simulink model "dc_motor"  (R2017b)
settings: Solver=VariableStepAuto  StartTime=0.0  StopTime=0.3  RelTol=1e-3
InitFcn:
  | before_simulation
values from neighbouring files (symbols this model uses):
  J = 0.08    [before_simulation.m]
  Kb = 0.87    [before_simulation.m]
  Kf = 0.043    [before_simulation.m]
  Km = 1.34    [before_simulation.m]
  L = 0.05    [before_simulation.m]
  R = 1.7    [before_simulation.m]
libraries: simulink_extras x6, simulink x4
settings Model: Creator=Iman  LastModifiedBy=Iman
settings DataIOCC: SaveFormat=Array

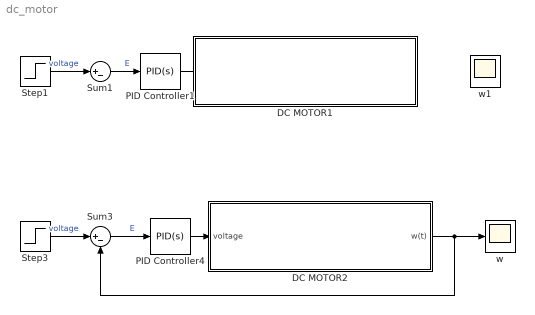
== system dc_motor ==
  DC MOTOR1 : Subsystem
  DC MOTOR2 : Subsystem
  PID Controller1 : simulink/Continuous/PID Controller  Controller=PID  TimeDomain=Continuous-time  SampleTime=-1  IntegratorMethod=Forward Euler  FilterMethod=Forward Euler  Form=Parallel  UseFilter=on  ControllerParametersSource=internal  P=89.3450380919849  I=457.97727460553  D=4.14027320331142  N=464.681776716059  InitialConditionSource=internal  InitialConditionForIntegrator=0  InitialConditionForFilter=0  ExternalReset=none  LimitOutput=off  UpperSaturationLimit=inf  LowerSaturationLimit=-inf  LinearizeAsGain=on  AntiWindupMode=none  Kb=1  TrackingMode=off  Kt=1  PParamMin=[]  PParamMax=[]  IParamMin=[]  IParamMax=[]  DParamMin=[]  DParamMax=[]  NParamMin=[]  NParamMax=[]  KbParamMin=[]  KbParamMax=[]  KtParamMin=[]  KtParamMax=[]  POutMin=[]  POutMax=[]  IOutMin=[]  IOutMax=[]  DOutMin=[]  DOutMax=[]  NOutMin=[]  NOutMax=[]  KbOutMin=[]  KbOutMax=[]  KtOutMin=[]  KtOutMax=[]  IntegratorOutMin=[]  IntegratorOutMax=[]  FilterOutMin=[]  FilterOutMax=[]  SumOutMin=[]  SumOutMax=[]  SumI1OutMin=[]  SumI1OutMax=[]  SumI2OutMin=[]  SumI2OutMax=[]  SumI3OutMin=[]  SumI3OutMax=[]  SumDOutMin=[]  SumDOutMax=[]  SaturationOutMin=[]  SaturationOutMax=[]  IntegratorContinuousStateAttributes=''  IntegratorStateMustResolveToSignalObject=off  IntegratorRTWStateStorageClass=Auto  FilterContinuousStateAttributes=''  FilterStateMustResolveToSignalObject=off  FilterRTWStateStorageClass=Auto  DifferentiatorICPrevScaledInput=0  DifferentiatorOutMin=[]  DifferentiatorOutMax=[]  InitialConditionSetting=State (most efficient)  FilterDiffOutCoefMin=[]  FilterDiffOutCoefMax=[]  SumDenOutMin=[]  SumDenOutMax=[]  SumNumOutMin=[]  SumNumOutMax=[]  ReciprocalOutMin=[]  ReciprocalOutMax=[]  DivideOutMin=[]  DivideOutMax=[]  TunerSelectOption=Transfer Function Based (PID Tuner App)
  PID Controller4 : simulink/Continuous/PID Controller  Controller=PID  TimeDomain=Continuous-time  SampleTime=-1  IntegratorMethod=Forward Euler  FilterMethod=Forward Euler  Form=Parallel  UseFilter=on  ControllerParametersSource=internal  P=89.3450380919849  I=457.97727460553  D=4.14027320331142  N=464.681776716059  InitialConditionSource=internal  InitialConditionForIntegrator=0  InitialConditionForFilter=0  ExternalReset=none  LimitOutput=off  UpperSaturationLimit=inf  LowerSaturationLimit=-inf  LinearizeAsGain=on  AntiWindupMode=none  Kb=1  TrackingMode=off  Kt=1  PParamMin=[]  PParamMax=[]  IParamMin=[]  IParamMax=[]  DParamMin=[]  DParamMax=[]  NParamMin=[]  NParamMax=[]  KbParamMin=[]  KbParamMax=[]  KtParamMin=[]  KtParamMax=[]  POutMin=[]  POutMax=[]  IOutMin=[]  IOutMax=[]  DOutMin=[]  DOutMax=[]  NOutMin=[]  NOutMax=[]  KbOutMin=[]  KbOutMax=[]  KtOutMin=[]  KtOutMax=[]  IntegratorOutMin=[]  IntegratorOutMax=[]  FilterOutMin=[]  FilterOutMax=[]  SumOutMin=[]  SumOutMax=[]  SumI1OutMin=[]  SumI1OutMax=[]  SumI2OutMin=[]  SumI2OutMax=[]  SumI3OutMin=[]  SumI3OutMax=[]  SumDOutMin=[]  SumDOutMax=[]  SaturationOutMin=[]  SaturationOutMax=[]  IntegratorContinuousStateAttributes=''  IntegratorStateMustResolveToSignalObject=off  IntegratorRTWStateStorageClass=Auto  FilterContinuousStateAttributes=''  FilterStateMustResolveToSignalObject=off  FilterRTWStateStorageClass=Auto  DifferentiatorICPrevScaledInput=0  DifferentiatorOutMin=[]  DifferentiatorOutMax=[]  InitialConditionSetting=State (most efficient)  FilterDiffOutCoefMin=[]  FilterDiffOutCoefMax=[]  SumDenOutMin=[]  SumDenOutMax=[]  SumNumOutMin=[]  SumNumOutMax=[]  ReciprocalOutMin=[]  ReciprocalOutMax=[]  DivideOutMin=[]  DivideOutMax=[]  TunerSelectOption=Transfer Function Based (PID Tuner App)
  Step1 : Step  Time=0  SampleTime=0.1
  Step3 : Step  Time=0  SampleTime=0.1
  Sum1 : Sum  Inputs=|+-
  Sum3 : Sum  Inputs=|+-
  w : Scope
  w1 : Scope
  wires:
  Sum3/1 -> PID Controller4/1  "E"
  Step3/1 -> Sum3/1  "voltage"
  PID Controller4/1 -> DC MOTOR2/1(voltage)
  DC MOTOR2/1(w(t)) -> w/1, Sum3/2
  ? -> w1/1, Sum1/2
  Step1/1 -> Sum1/1  "voltage"
  Sum1/1 -> PID Controller1/1  "E"
  PID Controller1/1 -> ?

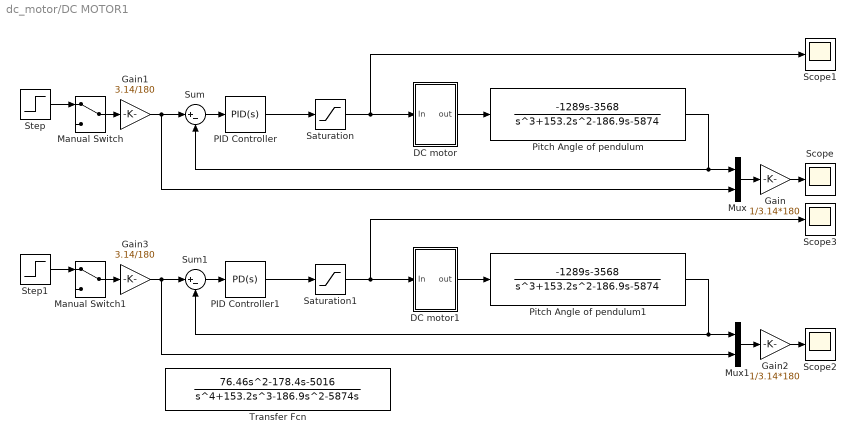
== system dc_motor/DC MOTOR1 ==
  DC motor : Subsystem
  DC motor1 : Subsystem
  Gain : Gain  Gain=1/3.14*180
  Gain1 : Gain  Gain=3.14/180
  Gain2 : Gain  Gain=1/3.14*180
  Gain3 : Gain  Gain=3.14/180
  Manual Switch : ManualSwitch
  Manual Switch1 : ManualSwitch
  Mux : Mux  Inputs=2
  Mux1 : Mux  Inputs=2
  PID Controller : simulink/Continuous/PID Controller  Controller=PID  TimeDomain=Continuous-time  SampleTime=-1  IntegratorMethod=Forward Euler  FilterMethod=Forward Euler  Form=Parallel  UseFilter=on  ControllerParametersSource=internal  P=-7.00083881462356  I=-74.399275138422  D=-0.163516565347945  N=4377.62555373868  InitialConditionSource=internal  InitialConditionForIntegrator=0  InitialConditionForFilter=0  ExternalReset=none  LimitOutput=off  UpperSaturationLimit=inf  LowerSaturationLimit=-inf  LinearizeAsGain=on  AntiWindupMode=none  Kb=1  TrackingMode=off  Kt=1  PParamMin=[]  PParamMax=[]  IParamMin=[]  IParamMax=[]  DParamMin=[]  DParamMax=[]  NParamMin=[]  NParamMax=[]  KbParamMin=[]  KbParamMax=[]  KtParamMin=[]  KtParamMax=[]  POutMin=[]  POutMax=[]  IOutMin=[]  IOutMax=[]  DOutMin=[]  DOutMax=[]  NOutMin=[]  NOutMax=[]  KbOutMin=[]  KbOutMax=[]  KtOutMin=[]  KtOutMax=[]  IntegratorOutMin=[]  IntegratorOutMax=[]  FilterOutMin=[]  FilterOutMax=[]  SumOutMin=[]  SumOutMax=[]  SumI1OutMin=[]  SumI1OutMax=[]  SumI2OutMin=[]  SumI2OutMax=[]  SumI3OutMin=[]  SumI3OutMax=[]  SumDOutMin=[]  SumDOutMax=[]  SaturationOutMin=[]  SaturationOutMax=[]  IntegratorContinuousStateAttributes=''  IntegratorStateMustResolveToSignalObject=off  IntegratorRTWStateStorageClass=Auto  FilterContinuousStateAttributes=''  FilterStateMustResolveToSignalObject=off  FilterRTWStateStorageClass=Auto  DifferentiatorICPrevScaledInput=0  DifferentiatorOutMin=[]  DifferentiatorOutMax=[]  InitialConditionSetting=State (most efficient)  FilterDiffOutCoefMin=[]  FilterDiffOutCoefMax=[]  SumDenOutMin=[]  SumDenOutMax=[]  SumNumOutMin=[]  SumNumOutMax=[]  ReciprocalOutMin=[]  ReciprocalOutMax=[]  DivideOutMin=[]  DivideOutMax=[]  TunerSelectOption=Transfer Function Based (PID Tuner App)
  PID Controller1 : simulink/Continuous/PID Controller  Controller=PD  TimeDomain=Continuous-time  SampleTime=-1  IntegratorMethod=Forward Euler  FilterMethod=Forward Euler  Form=Parallel  UseFilter=on  ControllerParametersSource=internal  P=-50.818900631766  I=-1096.43830658176  D=-2.68408169887524  N=33207.6857694086  InitialConditionSource=internal  InitialConditionForIntegrator=0  InitialConditionForFilter=0  ExternalReset=none  LimitOutput=off  UpperSaturationLimit=inf  LowerSaturationLimit=-inf  LinearizeAsGain=on  AntiWindupMode=none  Kb=1  TrackingMode=off  Kt=1  PParamMin=[]  PParamMax=[]  IParamMin=[]  IParamMax=[]  DParamMin=[]  DParamMax=[]  NParamMin=[]  NParamMax=[]  KbParamMin=[]  KbParamMax=[]  KtParamMin=[]  KtParamMax=[]  POutMin=[]  POutMax=[]  IOutMin=[]  IOutMax=[]  DOutMin=[]  DOutMax=[]  NOutMin=[]  NOutMax=[]  KbOutMin=[]  KbOutMax=[]  KtOutMin=[]  KtOutMax=[]  IntegratorOutMin=[]  IntegratorOutMax=[]  FilterOutMin=[]  FilterOutMax=[]  SumOutMin=[]  SumOutMax=[]  SumI1OutMin=[]  SumI1OutMax=[]  SumI2OutMin=[]  SumI2OutMax=[]  SumI3OutMin=[]  SumI3OutMax=[]  SumDOutMin=[]  SumDOutMax=[]  SaturationOutMin=[]  SaturationOutMax=[]  IntegratorContinuousStateAttributes=''  IntegratorStateMustResolveToSignalObject=off  IntegratorRTWStateStorageClass=Auto  FilterContinuousStateAttributes=''  FilterStateMustResolveToSignalObject=off  FilterRTWStateStorageClass=Auto  DifferentiatorICPrevScaledInput=0  DifferentiatorOutMin=[]  DifferentiatorOutMax=[]  InitialConditionSetting=State (most efficient)  FilterDiffOutCoefMin=[]  FilterDiffOutCoefMax=[]  SumDenOutMin=[]  SumDenOutMax=[]  SumNumOutMin=[]  SumNumOutMax=[]  ReciprocalOutMin=[]  ReciprocalOutMax=[]  DivideOutMin=[]  DivideOutMax=[]  TunerSelectOption=Transfer Function Based (PID Tuner App)
  Pitch Angle of pendulum : TransferFcn  Numerator="[-1289  -3568]"  Denominator="[1 153.2  -186.9  -5874]"  ContinuousStateAttributes='TETA'
  Pitch Angle of pendulum1 : TransferFcn  Numerator="[-1289  -3568]"  Denominator="[1 153.2  -186.9  -5874]"  ContinuousStateAttributes='TETA'
  Saturation : Saturate  UpperLimit=12  LowerLimit=-12
  Saturation1 : Saturate  UpperLimit=12  LowerLimit=-12
  Scope{,1..3} (4 alike) : Scope
  Step : Step  Time=0.001  Before=1  After=0  SampleTime=0.01
  Step1 : Step  Time=0.001  Before=1  After=0  SampleTime=0.01
  Sum : Sum  Inputs=|+-
  Sum1 : Sum  Inputs=|+-
  Transfer Fcn : TransferFcn  Numerator=[76.46 -178.4 -5016]  Denominator="[1 153.2  -186.9  -5874  0]"
  wires:
  DC motor/1(out) -> Pitch Angle of pendulum/1
  Sum/1 -> PID Controller/1
  PID Controller/1 -> Saturation/1
  Gain1/1 -> Mux/2, Sum/1
  Mux/1 -> Gain/1
  Gain/1 -> Scope/1
  Manual Switch/1 -> Gain1/1
  Step/1 -> Manual Switch/1
  Saturation/1 -> DC motor/1(In), Scope1/1
  Pitch Angle of pendulum/1 -> Sum/2, Mux/1
  Gain2/1 -> Scope2/1
  Mux1/1 -> Gain2/1
  Manual Switch1/1 -> Gain3/1
  DC motor1/1(out) -> Pitch Angle of pendulum1/1
  Step1/1 -> Manual Switch1/1
  Saturation1/1 -> DC motor1/1(In), Scope3/1
  Sum1/1 -> PID Controller1/1
  PID Controller1/1 -> Saturation1/1
  Gain3/1 -> Mux1/2, Sum1/1
  Pitch Angle of pendulum1/1 -> Sum1/2, Mux1/1

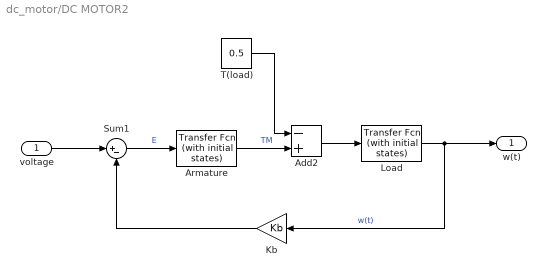
== system dc_motor/DC MOTOR2 ==
  voltage : Inport
  Add2 : Sum  Inputs=-+
  Armature : simulink_extras/Additional Linear/Transfer Fcn (with initial states)  N=[Km]  D=[L R]  X0=0
  Kb : Gain  Gain=Kb
  Load : simulink_extras/Additional Linear/Transfer Fcn (with initial states)  N=[1]  D=[J Kf]  X0=0
  Sum1 : Sum  Inputs=|+-
  T(load) : Constant  Value=0.5
  w(t) : Outport
  wires:
  Load/1 -> w(t)/1, Kb/1  "w(t)"
  Sum1/1 -> Armature/1  "E"
  voltage/1 -> Sum1/1
  Kb/1 -> Sum1/2
  T(load)/1 -> Add2/1
  Armature/1 -> Add2/2  "TM"
  Add2/1 -> Load/1

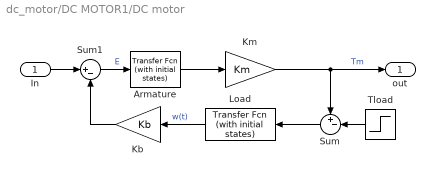
== system dc_motor/DC MOTOR1/DC motor ==
  In : Inport
  Armature : simulink_extras/Additional Linear/Transfer Fcn (with initial states)  N=[1]  D=[L R]  X0=0
  Kb : Gain  Gain=Kb
  Km : Gain  Gain=Km
  Load : simulink_extras/Additional Linear/Transfer Fcn (with initial states)  N=[1]  D=[J Kf]  X0=0
  Sum : Sum  Inputs=+-|
  Sum1 : Sum  Inputs=|+-
  Tload : Step  Time=0.2  After=0  SampleTime=0
  out : Outport
  wires:
  Load/1 -> Kb/1  "w(t)"
  In/1 -> Sum1/1
  Armature/1 -> Km/1
  Sum/1 -> Load/1
  Kb/1 -> Sum1/2
  Sum1/1 -> Armature/1  "E"
  Km/1 -> out/1, Sum/1  "Tm"
  Tload/1 -> Sum/2

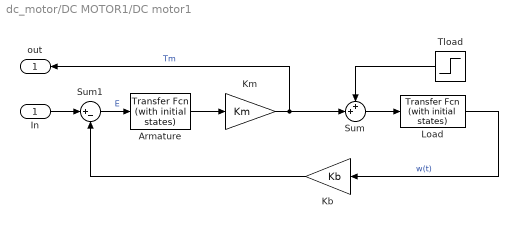
== system dc_motor/DC MOTOR1/DC motor1 ==
  In : Inport
  Armature : simulink_extras/Additional Linear/Transfer Fcn (with initial states)  N=[1]  D=[L R]  X0=0
  Kb : Gain  Gain=Kb
  Km : Gain  Gain=Km
  Load : simulink_extras/Additional Linear/Transfer Fcn (with initial states)  N=[1]  D=[J Kf]  X0=0
  Sum : Sum  Inputs=++|
  Sum1 : Sum  Inputs=|+-
  Tload : Step  Time=0.2  After=0  SampleTime=0
  out : Outport
  wires:
  Load/1 -> Kb/1  "w(t)"
  In/1 -> Sum1/1
  Tload/1 -> Sum/1
  Armature/1 -> Km/1
  Sum/1 -> Load/1
  Kb/1 -> Sum1/2
  Sum1/1 -> Armature/1  "E"
  Km/1 -> Sum/2, out/1  "Tm"
